simulink model "AccTarSel_PLAN_CTRL"  (R2018b)
settings: Solver=FixedStepDiscrete  StartTime=0.0  StopTime=inf  FixedStep=0.01  RelTol=1e-3
PostLoadFcn:
  | if any(exist('dsrtsu_mdlpostloadfcn', 'file') ~= 0), dsrtsu_mdlpostloadfcn('Execute', bdroot); end
undefined symbols (not defined in the file or in its folder): P_CutInEnable, P_dObjDrvOffMax, P_dObjDrvOffMin, P_dvarYMax4PO, P_dyCutInThres, P_kapHystThres, P_PlausIntegDisable, P_plausMin4PO, P_probExistMin4PO, P_StandObjEnable, P_tAxTrackNegLower, P_tAxTrackNegUpper, P_tAxTrackPosLower, P_tAxTrackPosUpper, P_tCurvFilt, P_tCutInFilt, P_tFiltAxAbsPONegFast, P_tFiltAxAbsPONegSlow, P_tFiltAxAbsPOPosFast, P_tFiltAxAbsPOPosSlow, P_tFiltAxAbsPOStand, P_tFiltVxAxPOFast, P_tFiltVxAxPOSlow, P_tMinDrvPhase, P_vObjDrvOff, P_vStandStill, P_vStandStillHyst, P_vyCutInThres
libraries: LPFilter x6, simulink x3
(part 3 of 3)

== system AccTarSel_PLAN_CTRL/ACC_Target_Selection/Subsystem/ValidObjCalc/TargetPlausCheck/Subsystem/CheckFOV ==
  note: logic to be expanded:
      | dx threshold can be adjusted regarding if current obj is already PO target
  In1 : Inport
  In2 : Inport  Port=2
  1-D Lookup Table : Lookup_n-D  NumberOfTableDimensions=1  LookupTableObject=''  BreakpointsForDimension1=[11.11,22.22]  BreakpointsForDimension1FirstPoint=10  BreakpointsForDimension2FirstPoint=10  BreakpointsForDimension1Spacing=12  BreakpointsForDimension2Spacing=12  IndexSearchMethod=Linear search  Table=[80,160]  ExtrapMethod=Clip  InternalRulePriority=Speed  RndMeth=Simplest  InputSameDT=on
  Bus Selector : BusSelector  OutputSignals=dx
  Bus Selector1 : BusSelector  OutputSignals=vRef
  Constant : Constant  Value=0  OutDataTypeStr=single
  Logical Operator : Logic  AllPortsSameDT=off  OutDataTypeStr=boolean
  Relational Operator : RelationalOperator  Operator=<=  OutDataTypeStr=boolean  RndMeth=Simplest
  Relational Operator1 : RelationalOperator  Operator=>  OutDataTypeStr=boolean  RndMeth=Simplest
  Out1 : Outport
  wires:
  In1/1 -> Bus Selector/1
  In2/1 -> Bus Selector1/1
  Bus Selector1/1 -> 1-D Lookup Table/1  "<vRef>"
  Bus Selector/1 -> Relational Operator1/1, Relational Operator/1  "<dx>"
  1-D Lookup Table/1 -> Relational Operator/2
  Constant/1 -> Relational Operator1/2
  Relational Operator1/1 -> Logical Operator/1
  Relational Operator/1 -> Logical Operator/2
  Logical Operator/1 -> Out1/1

== system AccTarSel_PLAN_CTRL/ACC_Target_Selection/Subsystem/ValidObjCalc/TargetPlausCheck/Subsystem/CheckMotSts ==
  note: MotionSts:
      | 0	Unknown
      | 1	Standstill
      | 2	Driving
      | 3	InvDriving
      | 4	Stopped
      | 5	InvStopped
  note: Type:
      | 0	Unknown
      | 1	Pedestrain
      | 2	Bi/Motor cycle
      | >=3	Vehicle
  In1 : Inport
  Bus Selector : BusSelector  OutputSignals=MotionSts,Type
  Constant : Constant  Value=2  OutDataTypeStr=single
  Constant1 : Constant  Value=4  OutDataTypeStr=single
  Constant2 : Constant  OutDataTypeStr=single
  Constant3 : Constant  Value=0  OutDataTypeStr=single
  Logical Operator1 : Logic  Operator=OR  Inputs=3  AllPortsSameDT=off  OutDataTypeStr=boolean
  Logical Operator2 : Logic  AllPortsSameDT=off  OutDataTypeStr=boolean
  P_StandObjEnable : Constant  Value=P_StandObjEnable  OutDataTypeStr=boolean
  Relational Operator : RelationalOperator  Operator===  OutDataTypeStr=boolean  RndMeth=Simplest
  Relational Operator1 : RelationalOperator  Operator===  OutDataTypeStr=boolean  RndMeth=Simplest
  Relational Operator2 : RelationalOperator  Operator===  OutDataTypeStr=boolean  RndMeth=Simplest
  Relational Operator3 : RelationalOperator  Operator=~=  OutDataTypeStr=boolean  RndMeth=Simplest
  Terminator : Terminator
  Out1 : Outport
  wires:
  In1/1 -> Bus Selector/1
  Bus Selector/1 -> Relational Operator2/1, Relational Operator1/1, Relational Operator/1  "<MotionSts>"
  Constant/1 -> Relational Operator/2
  Constant1/1 -> Relational Operator1/2
  Constant2/1 -> Relational Operator2/2
  Bus Selector/2 -> Relational Operator3/1  "<Type>"
  Constant3/1 -> Relational Operator3/2
  Relational Operator/1 -> Logical Operator1/1
  Relational Operator1/1 -> Logical Operator1/2
  Relational Operator2/1 -> Logical Operator1/3
  Logical Operator1/1 -> Logical Operator2/1
  Relational Operator3/1 -> Logical Operator2/2
  Logical Operator2/1 -> Out1/1
  P_StandObjEnable/1 -> Terminator/1

== system AccTarSel_PLAN_CTRL/ACC_Target_Selection/Subsystem/ValidObjCalc/TargetPlausCheck/Subsystem/CheckPlaus ==
  note: logic to be expanded:
      | plausibility threshold can be adjusted regarding if the current object is already PO target
  In1 : Inport
  P_plausMin4PO : Constant  Value=P_plausMin4PO  OutDataTypeStr=single
  Relational Operator1 : RelationalOperator  OutDataTypeStr=boolean  RndMeth=Simplest
  Out1 : Outport
  wires:
  In1/1 -> Relational Operator1/1
  P_plausMin4PO/1 -> Relational Operator1/2
  Relational Operator1/1 -> Out1/1

== system AccTarSel_PLAN_CTRL/ACC_Target_Selection/Subsystem/ValidObjCalc/CutInCalc/Subsystem/Subsystem/If Action Subsystem ==
  dy : Inport
  vy : Inport  Port=2
  Action Port : ActionPort  ActionType=then
  1-D Lookup Table : Lookup_n-D  NumberOfTableDimensions=1  LookupTableObject=''  BreakpointsForDimension1=[0.5,1.5]  BreakpointsForDimension1FirstPoint=10  BreakpointsForDimension2FirstPoint=10  BreakpointsForDimension1Spacing=12  BreakpointsForDimension2Spacing=12  IndexSearchMethod=Linear search  Table=[0,1.5]  ExtrapMethod=Clip  InternalRulePriority=Speed  RndMeth=Simplest  InputSameDT=on
  1-D Lookup Table1 : Lookup_n-D  NumberOfTableDimensions=1  LookupTableObject=''  BreakpointsForDimension1=[1,1.8]  BreakpointsForDimension1FirstPoint=10  BreakpointsForDimension2FirstPoint=10  BreakpointsForDimension1Spacing=12  BreakpointsForDimension2Spacing=12  IndexSearchMethod=Linear search  Table=[1,0]  ExtrapMethod=Clip  InternalRulePriority=Speed  RndMeth=Simplest  InputSameDT=on
  Abs : Abs
  Abs1 : Abs
  Add : Sum
  Constant : Constant  Value=0  OutDataTypeStr=single
  Max : MinMax  Function=max  Inputs=2
  Max1 : MinMax  Inputs=2
  Multiply : Product
  Switch : Switch  Criteria=u2 > Threshold
  Out1 : Outport
  Out2 : Outport  Port=2
  wires:
  vy/1 -> Multiply/1, Abs1/1
  1-D Lookup Table/1 -> Multiply/2  "tPred"
  dy/1 -> Switch/2, Add/1
  Multiply/1 -> Add/2
  Add/1 -> Max1/2, Max/1
  Constant/1 -> Max1/1, Max/2
  Switch/1 -> Out2/1, Abs/1  "dyPred"
  1-D Lookup Table1/1 -> Out1/1
  Abs/1 -> 1-D Lookup Table1/1
  Abs1/1 -> 1-D Lookup Table/1
  Max/1 -> Switch/1
  Max1/1 -> Switch/3

== system AccTarSel_PLAN_CTRL/ACC_Target_Selection/Subsystem/ValidObjCalc/CutInCalc/Subsystem/Subsystem/If Action Subsystem1 ==
  dy : Inport
  Action Port : ActionPort  ActionType=else
  Constant : Constant  Value=0  OutDataTypeStr=single
  Out1 : Outport
  Out2 : Outport  Port=2
  wires:
  Constant/1 -> Out1/1
  dy/1 -> Out2/1

== stateflow chart AccTarSel_PLAN_CTRL/ACC_State_Machine1 ==
  note: MainState
      | 0	OFF
      | 1	PASSIVE
      | 2	ACTIVE_Drive
      | 3	ACTIVE_Standstill
      | 4	OVERRIDE
  state OFF
    en:
    AST_Info_st.MainState = 0;
    AST_Info_st.tMinInDrv = 0;
    AST_Info_st.vSet = 0;
  state OVERRIDE
    en:
    AST_Info_st.MainState = 4;
    AST_Info_st.tMinInDrv = 0;
  state PASSIVE
    en:
    AST_Info_st.MainState = 1;
    AST_Info_st.tMinInDrv = 0;
  state ACTIVE
    en:
    if ((NET_DrvAction_st.ACC_SetSw == 1)&&(NET_DrvAction_st.ACC_SetSwK1 == 0))
    AST_Info_st.vSet = round(VSI_VehState_st.vRef*1.05*3.6)/1.05/3.6;
    end
    AST_Info_st.vSet = min(AST_Info_st.vSet, (120/1.05)/3.6);
    AST_Info_st.vSet = max(AST_Info_st.vSet, (30/1.05)/3.6);
    du:
    if ((NET_DrvAction_st.ACC_SpdIncSw == 1)&&(NET_DrvAction_st.ACC_SpdIncSwK1 == 0))
    AST_Info_st.vSet = AST_Info_st.vSet + (5 - mod(round(AST_Info_st.vSet*1.05*3.6),5))/1.05/3.6;
    else if ((NET_DrvAction_st.ACC_SpdDecSw == 1)&&(NET_DrvAction_st.ACC_SpdDecSwK1 == 0))
    AST_Info_st.vSet = AST_Info_st.vSet + (mod(5 - mod(round(AST_Info_st.vSet*1.05*3.6),5),5))/1.05/3.6 - 5/1.05/3.6;
    end
    end
    if (vSet_HMI.vSetAccSpd ~= 0)
    AST_Info_st.vSet = vSet_HMI.vSetAccSpd/1.05/3.6;
    end
    AST_Info_st.vSet = min(AST_Info_st.vSet, (120/1.05)/3.6);
    AST_Info_st.vSet = max(AST_Info_st.vSet, (30/1.05)/3.6);
    state Drive
      en:
      AST_Info_st.MainState = 2;
      du:
      if(VSI_VehState_st.vRef > P_vStandStillHyst)
      if(AST_Info_st.tMinInDrv > SYS_Info_st.dT)
      AST_Info_st.tMinInDrv = AST_Info_st.tMinInDrv - SYS_Info_st.dT;
      else
      AST_Info_st.tMinInDrv = 0;
      end
      end
    state Standstill
      en:
      AST_Info_st.MainState = 3;
      AST_Info_st.tMinInDrv = P_tMinDrvPhase;
    (default) -> Drive
    Drive -> Standstill : [VSI_VehState_st.vRef < P_vStandStill...
        | &&AST_Info_st.tMinInDrv == 0]
    Standstill -> Drive : [DrvOffEnable == 1]
  (default) -> OFF
  OVERRIDE -> OFF [order 3] : [NET_DrvAction_st.ACC_MainSw == 0]
  ACTIVE -> OFF [order 3] : [NET_DrvAction_st.ACC_MainSw == 0]
  OVERRIDE -> PASSIVE [order 2] : [NET_DrvAction_st.ACC_CancelSw == 1||NET_DrvAction_st.BrakePedalApply == 1||NET_DrvAction_st.GearLever < 3]
  ACTIVE -> OVERRIDE [order 1] : [NET_DrvAction_st.DrvOverride == 1]
  OVERRIDE -> ACTIVE [order 1] : [NET_DrvAction_st.DrvOverride == 0]
  OFF -> PASSIVE : [NET_DrvAction_st.ACC_MainSw == 1]
  PASSIVE -> OFF [order 2] : [NET_DrvAction_st.ACC_MainSw == 0]
  PASSIVE -> ACTIVE [order 1] : [(NET_DrvAction_st.ACC_SetSw == 1||(NET_DrvAction_st.ACC_ResSw == 1&&AST_Info_st.vSet ~= 0))&&NET_DrvAction_st.BrakePedalApply == 0&&NET_DrvAction_st.GearLever >= 3]
  ACTIVE -> PASSIVE [order 2] : [NET_DrvAction_st.ACC_CancelSw == 1||NET_DrvAction_st.BrakePedalApply == 1||NET_DrvAction_st.GearLever < 3]
  data: NET_DrvAction_st input; AST_Info_st output Bus: AST_INFO_ST; VSI_VehState_st input; DrvOffEnable input; SYS_Info_st input; P_tMinDrvPhase input; P_vStandStill input; P_vStandStillHyst input; vSet_HMI input Bus: ACC_HMI_REQ

== matlab function AccTarSel_PLAN_CTRL/Choose Polynominal/Polynominal/Polynominal_Solver ==
  data: MINT_V input; a_des output; DT input; MAXT_V input; MINT input; MAXT input; SET_SPEED input; DV input; DS input; v_f input; a_f input; v_ego input; a_ego input; KJ input; KT input; KDS input; KJV input; KTV input; KDSV input; MAX_ACC input; MIN_ACC input; speed_limit input; aDesIndex input; v_des output; dist input
function [a_des,v_des] = ACC_PLANNING(MINT_V,DT,MAXT_V, MINT,MAXT,SET_SPEED,DV,DS,v_f,a_f,v_ego,a_ego,KJ,KT,KDS,KJV, KTV, KDSV,MAX_ACC, MIN_ACC,speed_limit,aDesIndex,...
    dist)

        s_of_t = zeros(200,1);
        v_of_t = zeros(200,1);
        a_of_t = zeros(200,1);
        t_data = zeros(200,1);
        a_des = 0;
        v_des = 0;
        
    if dist >= 100

        [cost_graph] = cal_velocity_control(MINT_V,DT,MAXT_V, SET_SPEED,DV,v_ego, a_ego, KJV, KTV, KDSV); 
        [cost_optimal] = check_quantic_status(cost_graph,speed_limit, MAX_ACC, MIN_ACC,MAXT_V); 
        [s_of_t, v_of_t,a_of_t, t_data] = combination_quantic(cost_optimal); 
        a_des = min(max(a_of_t(aDesIndex),-1.5),1.5);
        v_des = min(max(v_of_t(2),0),speed_limit);
        
    else
        D0 = 0; % ONLY for test convenience
        TTC = 0;
        
        [cost_graph] = cal_distance_control(MINT,DT,MAXT,v_f,a_f,dist,D0,TTC,DS,v_ego,a_ego,KJ,KT,KDS);
        cost_optimal = check_status(cost_graph,speed_limit, MAX_ACC, MIN_ACC,MAXT);
        [s_of_t, v_of_t,a_of_t, t_data] = combination_quintic(cost_optimal);
        a_des = min(max(a_of_t(aDesIndex),-4),1.5);
        v_des = min(max(v_of_t(2),0),speed_limit);
    end
    
end


    


function [cost_graph] = cal_distance_control(MINT,DT,MAXT,v_f,a_f,dist,D0,TTC,DS,v_pre,a_pre,KJ,KT,KDS)
    
    cost_graph = ones(400,12)* 500; 
    index = 1;
    for Ti = MINT : DT : MAXT
        v_f_t = cal_v_f_t(v_f, a_f, Ti);
        dist_t = cal_dist_t(dist,v_f,a_f,Ti);
        [s_des] = cal_s_des(D0, TTC, v_f_t);
        [s_target] = cal_s_target(s_des,dist_t);
        [s_target_d] = cal_s_target_d(v_f_t, TTC, a_f);
        [s_target_dd] = cal_s_target_dd(a_f);
        delta_s = 0.1 * s_target;
        
        for Si = (s_target - delta_s) : DS : (s_target + delta_s) 
            s0 = 0;
            v0 = v_pre;
            a0 = a_pre;
            se = Si;
            ve = s_target_d;
            ae = s_target_dd;
            [a0, a1, a2, a3, a4,a5] = quintic_polynomial(s0, ...
                v0, a0, se, ve, ae,Ti);
            %get the quintic polu parameters;
            [jerk,count] = cal_jerk(a3,a4,a5,Ti);
            cost_J = mean(abs(jerk(1:count)));
            cost_T = Ti;
            cost_DS = sqrt((s_target - Si)^2);
            cost_total = KJ * cost_J + KT * cost_T + KDS * cost_DS;
            cost_graph(index,:) = [cost_total,Ti,Si,cost_J,cost_T,cost_DS,...
                a0, a1, a2, a3, a4, a5];
            
            index = index + 1;
        end
    end
    cost_graph = sortrows(cost_graph);
end

function [cost_graph] = cal_velocity_control(MINT_V,DT,MAXT_V, SET_SPEED,DV,v_pre, a_pre, KJV, KTV, KDSV)
    cost_graph = ones(400,11)* 500;    
    index = 1;
    delta_v = 0.1 * SET_SPEED;

    for Ti = MINT_V : DT : MAXT_V
        for Ve = SET_SPEED - 3 : DV : SET_SPEED + 3
            s0 = 0;
            v0 = v_pre;
            a0 = a_pre;
            ve = Ve;
            ae = 0;
            [a0, a1, a2, a3, a4] = quantic_polynomial(s0, ...
                v0, a0, ve, ae,Ti);
            [jerk,count] = cal_quantic_jerk(a3,a4,Ti);
            cost_J = mean(abs(jerk(1:count)));
            cost_T = Ti;
            cost_DV = sqrt((SET_SPEED - Ve)^2);
            cost_total = KJV * cost_J + KTV * cost_T + KDSV * cost_DV;
            cost_graph(index,:) = [cost_total,Ti,Ve,cost_J,cost_T,cost_DV,...
                a0, a1, a2, a3, a4];

            index = index + 1;
        end
    end
    cost_graph = sortrows(cost_graph);
end

function [cost_optimal] = check_status(cost_graph,speed_limit, MAX_ACC, MIN_ACC,MAXT)
    i = 1;
    COND = 1;
    cost_optimal = zeros(1,12);
    LEN_T = 0;
    
    if isempty(cost_graph)
        cost_optimal=  zeros(1,12);
        fprintf("error in cost graph.");
        return;
    end
    
    valid_range = find(cost_graph(:,2) == 500);
    valid_size = valid_range(1);
    
    while COND == 1
        

        
        poly_para = cost_graph(i,7:12);
        a0 = poly_para(1); a1 = poly_para(2); a2 = poly_para(3); 
        a3 = poly_para(4); a4 = poly_para(5); a5 = poly_para(6);
        
        Te = cost_graph(i,2);
        LEN_T = double(Te * 5 + 1);
        vt = zeros(200,1);
        at = zeros(200,1);
        
        
        for j = 1: LEN_T
            t = (j-1) * 0.2;
            vt(j) = calc_first_derivative(a1,a2,a3,a4,a5,t);
            at(j) =  calc_second_derivative(a2,a3,a4,a5,t);
        end
        
        if cost_graph(i,1) == 500
            COND = 2;
        end
        
        
        
        
        if (max(abs(vt)) <= speed_limit && max(at) <= MAX_ACC && min(at) >= MIN_ACC)
            cost_optimal = cost_graph(i,:);
            COND = 2;
        end
        
        i = i + 1;
        
        if i == valid_size
            COND = 2;
            POS = find(cost_graph(:,2) == MAXT);
            POS_first = POS(1); % find the first combination with longest T; 
            cost_optimal = cost_graph(POS_first,:);
        end
    end
end

function [cost_optimal] = check_quantic_status(cost_graph,speed_limit, MAX_ACC, MIN_ACC,MAXT_V)
    i = 1;
    COND = 1;
    cost_optimal = zeros(1,11);
    LEN_T = 0;
    
    if isempty(cost_graph)
        cost_optimal=  zeros(1,11);
        fprintf("error in cost graph.");
        return;
    end
    
    valid_range = find(cost_graph(:,2) == 500);
    valid_size = valid_range(1);

    while COND == 1

        
        poly_para = cost_graph(i,7:11);
        a0 = poly_para(1); a1 = poly_para(2); a2 = poly_para(3); 
        a3 = poly_para(4); a4 = poly_para(5); 
        
        Te = cost_graph(i,2);
        
        LEN_T = double(Te * 5 + 1);
        vt = zeros(200,1);
        at = zeros(200,1);
        
        for j = 1: LEN_T
            t = (j-1) * 0.2;
            vt(j) = calc_quantic_first_derivative(a1,a2,a3,a4,t);
            at(j) = calc_quantic_second_derivative(a2,a3,a4,t);
        end
        
        
        if cost_graph(i,1) == 500
            COND = 2;
        end
        
        if (max(abs(vt)) <= speed_limit && max(at) <= MAX_ACC && min(at) >= MIN_ACC)
            cost_optimal(1:11) = cost_graph(i,:);
            COND = 2;
        end
        
        i = i + 1;
        
        if i == valid_size
            COND = 2;
            POS = find(cost_graph(:,2)==MAXT_V);
            POS_first = POS(1); % find the first combination with longest T; 
            cost_optimal(1:11)  = cost_graph(POS_first,:);
        end
    end
end

function [a0, a1, a2, a3, a4] = quantic_polynomial(xs, ...
    vxs, axs, vxe, axe,T)
    
    A  =[1,0,0,0,0;0,1,0,0,0;0,0,2,0,0;...
        0,1,2*T,3*T^2,4*T^3;0,0,2,6*T,12*T^2];
    
    if det(A) == 0
        a0 = [];
        a1 = [];
        a2 = [];

        a3 = [];
        a4 = [];


        fprintf('cannot calculate quintic polynomial paras.');
        return;
    end
    
    
    b = [xs,vxs,axs,vxe,axe]';
    x = pinv(A) * b;
    
    a0 = x(1);
    a1 = x(2);
    a2 = x(3);
    a3 = x(4);
    a4 = x(5);
end

function [a0, a1, a2, a3, a4,a5] = quintic_polynomial(xs, ...
    vxs, axs, xe, vxe, axe,T)
% A = [0,0,0,0,0,1; T^5,T^4,T^3,T^2,T,1;...
%     0,0,0,0,1,0 ; 5*T^4  4*T^3 3*T^2 2*T 1 0 ; ...
%     0 0 0 2 0 0; 20*T^3 12*T^2 6*T 2 0 0];
% b = [xs, xe, vxs, vxe, axs, 0]';
% x = A\b;
% a5 = x(1);
% a4 = x(2);
% a3 = x(3);
% a2 = x(4);
% a1 = x(5);
% a0 = x(6);
A = [T^3 T^4 T^5; 3*T^2 4*T^3 5*T^4; 6*T 12*T^2 20*T^3];
b = [(xe - xs  - vxs*T - 0.5*axs*T^2); (vxe- vxs - axs*T ); (axe - axs)];

if det(A) == 0
    a0 = [];
    a1 = [];
    a2 = [];

    a3 = [];
    a4 = [];
    a5 = [];  
    
    fprintf('cannot calculate quintic polynomial paras.');
    return;
end


    
    
x = pinv(A) * b;
a0 = xs;
a1 = vxs;
a2 = axs/2;

a3 = x(1);
a4 = x(2);
a5 = x(3);
end

function [jerk,count] = cal_jerk(a3,a4,a5,Ti)
    seg = 8 / 0.1 + 1;
    count = Ti / 0.1 + 1;
    index = 1;
    jerk = zeros(1,seg);
    
    for k = 1:seg
        i  = k * 0.1;
        jerk(index) =  6* a3  + 24 * a4 * i + 60* a5 *i^2;
        index = index + 1;
    end
end

function [jerk,count] = cal_quantic_jerk(a3,a4,Ti)
    seg = 8 / 0.1 + 1;
    count = Ti / 0.1 + 1;
    index = 1;
    jerk = zeros(1,seg);
    
    for k = 1:seg
        i  = k * 0.1;
        jerk(index) =  6* a3 + 24 * a4 * i;
        index = index + 1;
    end
end

function [s_of_t, v_of_t,a_of_t, t_data] = combination_quintic(cost_optimal)
    if isempty(cost_optimal)
        s_of_t = zeros(200,1);
        v_of_t = zeros(200,1);
        t_data = zeros(200,1);
        fprintf("error in optimal cost graph.");
        return;
    end

   
    Te = cost_optimal(2);
    poly_para = cost_optimal(7:12);
    a0 = poly_para(1); a1 = poly_para(2); a2 = poly_para(3); 
    a3 = poly_para(4); a4 = poly_para(5); a5 = poly_para(6);
   s_of_t = zeros(200,1);
    v_of_t = zeros(200,1);
    a_of_t = zeros(200,1);
    t_data = zeros(200,1);
    
    index = 1;
    seg = Te / 0.1 - 1;
    
    for i = 0 : seg
        t = i * 0.1;
        s_of_t(index) = calc_point(a0,a1,a2,a3,a4,a5,t);
        v_of_t(index) = calc_first_derivative(a1,a2,a3,a4,a5,t);
        a_of_t(index) =  calc_second_derivative(a2,a3,a4,a5,t);
        t_data(index) = t;
        index = index + 1;
    end
end

function [s_of_t, v_of_t,a_of_t,t_data] = combination_quantic(cost_optimal)
    if isempty(cost_optimal)

        fprintf("error in optimal cost graph.");
        return;
    end

    Te = cost_optimal(2);
    poly_para = cost_optimal(7:11);
    a0 = poly_para(1); a1 = poly_para(2); a2 = poly_para(3); 
    a3 = poly_para(4); a4 = poly_para(5); 
    s_of_t = zeros(200,1);
    v_of_t = zeros(200,1);
    a_of_t = zeros(200,1);
    t_data = zeros(200,1);
    
    index = 1;
    seg = Te / 0.1 - 1;
    
    for i = 0 : seg
        t = i * 0.1;
        s_of_t(index) = cal_quantic_point(a0,a1,a2,a3,a4,t);
        v_of_t(index) = calc_quantic_first_derivative(a1,a2,a3,a4,t);
        a_of_t(index) = calc_quantic_second_derivative(a2,a3,a4,t);
        t_data(index) = t;
        index = index + 1;
    end
end


function [xt] = calc_point(a0,a1,a2,a3,a4,a5,T)
    xt = a0 + a1 * T + a2 * T^2 + a3 * T^3 + a4 * T^4 + a5 * T^5;
end

function [xt] = cal_quantic_point(a0,a1,a2,a3,a4,T)
    xt = a0 + a1 * T + a2 * T^2 + a3 * T^3 + a4 * T^4;
end

function [xt] =calc_first_derivative(a1,a2,a3,a4,a5,t)
xt = a1 + 2 * a2 * t + 3 * a3 * t^2 + 4 * a4 * t^3 + 5 * a5 * t^4;
end

function [xt]  = calc_second_derivative(a2,a3,a4,a5,t)
xt = 2* a2 + 6* a3 * t + 12 * a4 * t^2 + 20* a5 *t^3;
end

function [xt] =calc_quantic_first_derivative(a1,a2,a3,a4,t)
xt = a1 + 2 * a2 * t + 3 * a3 * t^2 + 4 * a4 * t^3;
end

function [xt]  = calc_quantic_second_derivative(a2,a3,a4,t)
xt = 2* a2 + 6* a3 * t + 12 * a4 * t^2;
end

function v_f_t = cal_v_f_t(v_f, a_f, Ti)
    %calculate v_f of time.
    v_f_t = v_f + a_f * Ti;
end

function dist_t = cal_dist_t(dist,v_f,a_f,Ti)
    %calculate distance of time.
    dist_t = dist + v_f * Ti + 1/2 * a_f * Ti^2;
end


function [s_des] = cal_s_des(D0, TTC, v_f_t)
    %calculate desired s.
%     s_des = D0 + TTC * v_f_t;
     s_des = 20; % here we made a simplification
end


function [s_target] = cal_s_target(s_des,dist_t)
    %calculate s target.
    s_target = dist_t - s_des;
end

function [s_target_d] = cal_s_target_d(v_f_t, TTC, a_f)
    %calculate v_f of time.
%     s_target_d = v_f_t - TTC * a_f;
    s_target_d = v_f_t; % here we made a simplification
end


function [s_target_dd] = cal_s_target_dd(a_f)
    s_target_dd = a_f;
end

== matlab function AccTarSel_PLAN_CTRL/Choose Exponential/Exponential/Subsystem/If Action Subsystem/exponential_Solver ==
  data: vSet input; T0 output; vEgoInit input; aEgoInit input; T1 output; T2 output
function [T0,T1,T2] = fcn(vSet,vEgoInit,aEgoInit)
dt = 0.2;
t = 0:dt:13;
dTarget = 10;
vt = 0;


tTarget = 8;
TimeGap = 2;

index = 1;

T0Array = zeros(1,256);
T1Array = zeros(1,256);
T2Array = zeros(1,256);
maxA = zeros(1,256);
%tConverg = zeros(1,256);
vDiffAtSetTime = zeros(1,256);
vDiffAtFinal = zeros(1,256);
for T0= 1:0.2:4
    for T1 = 0.5:0.5
        for T2 = 1:0.2:4

            %vEgo = zeros(1,length(t));
            %vEgo(1) = vEgoInit;
            %vxAbs = zeros(1,length(t));
            %vx = zeros(1,length(t));
            %aCmd  = zeros(1,length(t));
            %d = zeros(1,length(t));
            %deltaD = zeros(1,length(t));
            
            %deltaV = aEgoInit * T2;
            %vProfile = 0;
            %vx(1) = deltaV + vProfile;
            %vxAbs(1) = vx(1) + vEgo(1);
            %vDiff = zeros(1,length(t));
            %dx = 0;
            %dAim = 0;
            %tConvergence = 255;
            
	if 0
%             for i = 1:length(t)-1                
%                 deltaD(i) = dAim-dx;
%                 vProfile = deltaD(i)/T1;
%                 deltaV = vx(i) - vProfile;
%                 aCmd(i) = deltaV/T2;
%                 [d(i+1),vEgo(i+1)] = StateSpace(d(i),vEgo(i),aCmd(i),dt);
%                 
%                 kf = dt/T0;
%                 vxAbs(i+1) = (1-kf)*vxAbs(i) + kf*vSet;
%                 vx(i+1) = vxAbs(i+1) - vEgo(i+1);
%                 
%                 if (abs(vEgo(i+1) - vSet) < 0.277)&&(tConvergence == 255)
%                     tConvergence = i*dt;
%                 end
%                vDiff(i) = vSet - vEgo(i);
% 
%             end
%             aMax = max(abs(aCmd));
%             vDiffAtSetT = vDiff(tTarget/dt);
%             vDiffAtF = vDiff(end-1);
    else
            vAim0 = aEgoInit * T2 + vEgoInit;
            %vAim = (vAim0 - vSet)*exp(-t/T0) + vSet;
            if T0 == T2
                T0Act = T0 - dt;
                T2Act = T2 + dt;
            else
                T0Act = T0;
                T2Act = T2;
            end
            C1 = (vAim0-vSet)/(1-T2Act/T0Act);
            C2 = vEgoInit - C1 - vSet;
            Tstart = 0;
            Tend = 13;
            %[tConvergence,vThres] = BiSearch(C1,C2,T0Act,T2Act,vSet,vEgoInit,Tstart,Tend);
            
            aMax = max(abs(calcAEgo(C1,C2,T0Act,T2Act,t)));
            vDiffAtSetT = vSet - calcVEgo(C1,C2,T0Act,T2Act,vSet,tTarget);
            vDiffAtF = vSet - calcVEgo(C1,C2,T0Act,T2Act,vSet,13);
    end
%             RG(index).deltaD = deltaD;
%             RG(index).aCmd = aCmd;
%             RG(index).d = d;
%             RG(index).vEgo = vEgo;  
%             RG(index).vxAbs = vxAbs;  
%             RG(index).vx = vx; 
            T0Array(index) = T0;
            T1Array(index) = T1;
            T2Array(index) = T2;
            %tConverg(index) = min(5,abs(tConvergence-tTarget));
            maxA(index) = min(2,abs(aMax));
            vDiffAtSetTime(index) = min(4,abs(vDiffAtSetT));
            vDiffAtFinal(index) = min(1,abs(vDiffAtF));
            index = index + 1;

        end
    end
end


% figure
% plot(maxDeltaD)
% hold on
% plot(tConverg)
% plot(maxA)

%kT = interp1([0,5],[1,0.05],tConverg,'linear');
kA = interp1([0,3],[1,0.05],maxA,'linear');
kVdiff = interp1([0,2],[1,0.05],vDiffAtSetTime,'linear');
kVdiffF = interp1([0,1],[1,0.05],vDiffAtFinal,'linear');
k = (0.8*kVdiff + 0.2*kVdiffF).*kA;

[maxK,imax] = max(k);
minK = min(k);
if maxK == minK
    T0 = 2;
    T1 = 2;
    T2 = 2;
else
    T0 = T0Array(imax);
    T1 = T1Array(imax);
    T2 = T2Array(imax);
end

end
%%
% function [d_k, v_k] = StateSpace(d_k_pre, v_k_pre,a_des, dt)    
%     d_k = d_k_pre + dt * v_k_pre + 0.5 * dt^2 * a_des;
%     v_k = v_k_pre + dt * a_des; 
% end
%%
function [vEgo] = calcVEgo(C1,C2,T0,T2,vSet,t)
    vEgo = C1*exp(-t/T0) + C2*exp(-t/T2) + vSet;
end

function [aEgo] = calcAEgo(C1,C2,T0,T2,t)
    aEgo = -(C1/T0)*exp(-t/T0) - (C2/T2)*exp(-t/T2);
end
    
function [tConvergence,vThres] = BiSearch(C1,C2,T0,T2,vSet,vEgoInit,Tstart,Tend)
    if vSet > vEgoInit
        epsilon = -0.27;
    else
        epsilon = 0.27;
    end

    vStart = calcVEgo(C1,C2,T0,T2,vSet,Tstart) - (vSet + epsilon);
    vEnd = calcVEgo(C1,C2,T0,T2,vSet,Tend) - (vSet + epsilon);
    SignStart = sign(vStart);
    SignEnd = sign(vEnd);
    vThres = vSet + epsilon;

    if SignStart ~= SignEnd
        %find convergence point
        vFind = 255;
        count = 1;
        while ((abs(vFind) > 0.05)&&(count < 10))
            tFind = (Tstart + Tend)/2;
            vFind = calcVEgo(C1,C2,T0,T2,vSet,tFind) - (vSet + epsilon);
            SignFind = sign(vFind);
            if SignFind == SignStart
                Tstart = tFind;
            else
                Tend = tFind;
            end
            count = count + 1;
            tConvergence = tFind;
        end
    else
        tConvergence = 255;
    end
end
